simulink library "WellClearMetricsBlock"  (R2018b)
settings: Solver=VariableStepAuto  StartTime=0.0  StopTime=10.0  RelTol=1e-3
undefined symbols (not defined in the file): magnitude, wcm_altThresh, wcm_HMD, wcm_modTau, wcm_rangeThresh, wcm_TOCA
libraries: simulink x3
settings Model: Creator=BI28030  LastModifiedBy=BI28030

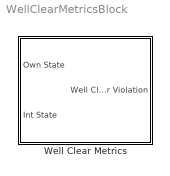
== system WellClearMetricsBlock ==
  Well Clear Metrics : Subsystem  mask{tauThreshold=wcm_modTau, hmdThreshold=wcm_HMD, tauVThreshold=wcm_TOCA, altThreshold=wcm_altThresh, rngThreshold=wcm_rangeThresh}
      mask prompts: tauThreshold "Modified Tau Threshold (s)"; hmdThreshold "Horizontal Miss Distance Threshold (ft)"; tauVThreshold "Time to Co-Altitude Threshold (s)"; altThreshold "Altitude Threshold (ft)"; rngThreshold "Range Threshold (ft)"
      mask help: Determines whether the intruder aircraft is within the bounds of a tau-based well clear region. Input is ownship and intruder 6-element state vectors in north, east, altitude coordinates. Returns true if a well-clear violation exists, false otherwise.

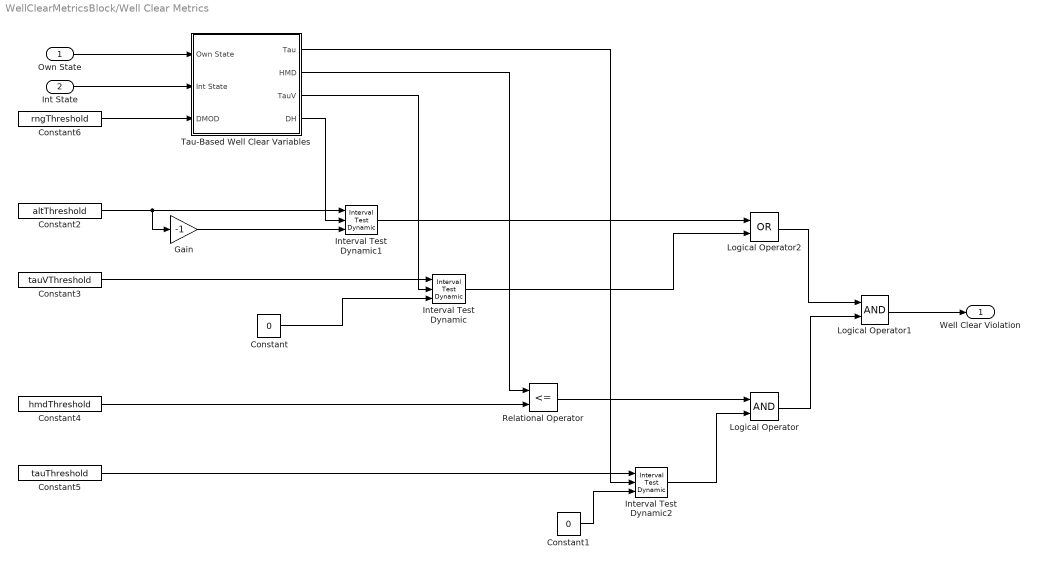
== system WellClearMetricsBlock/Well Clear Metrics ==
  Own State : Inport
  Int State : Inport  Port=2
  Constant : Constant  Value=0
  Constant1 : Constant  Value=0
  Constant2 : Constant  Value=altThreshold
  Constant3 : Constant  Value=tauVThreshold
  Constant4 : Constant  Value=hmdThreshold
  Constant5 : Constant  Value=tauThreshold
  Constant6 : Constant  Value=rngThreshold
  Gain : Gain  Gain=-1
  Interval Test Dynamic : simulink/Logic and Bit Operations/Interval Test Dynamic  IntervalClosedRight=on  IntervalClosedLeft=on  OutDataTypeStr=boolean
      settings: SourceProductName=Simulink  SourceProductBaseCode=SL
  Interval Test Dynamic1 : simulink/Logic and Bit Operations/Interval Test Dynamic  IntervalClosedRight=on  IntervalClosedLeft=on  OutDataTypeStr=boolean
      settings: SourceProductName=Simulink  SourceProductBaseCode=SL
  Interval Test Dynamic2 : simulink/Logic and Bit Operations/Interval Test Dynamic  IntervalClosedRight=on  IntervalClosedLeft=on  OutDataTypeStr=boolean
      settings: SourceProductName=Simulink  SourceProductBaseCode=SL
  Logical Operator : Logic  AllPortsSameDT=off  OutDataTypeStr=boolean
  Logical Operator1 : Logic  AllPortsSameDT=off  OutDataTypeStr=boolean
  Logical Operator2 : Logic  Operator=OR  AllPortsSameDT=off  OutDataTypeStr=boolean
  Relational Operator : RelationalOperator  Operator=<=  OutDataTypeStr=boolean  RndMeth=Nearest
  Tau-Based Well Clear Variables : Subsystem
  Well Clear Violation : Outport
  wires:
  Tau-Based Well Clear Variables/4(DH) -> Interval Test Dynamic1/2
  Tau-Based Well Clear Variables/3(TauV) -> Interval Test Dynamic/2
  Tau-Based Well Clear Variables/2(HMD) -> Relational Operator/1
  Relational Operator/1 -> Logical Operator/1
  Constant/1 -> Interval Test Dynamic/3
  Constant3/1 -> Interval Test Dynamic/1
  Int State/1 -> Tau-Based Well Clear Variables/2(Int State)
  Constant2/1 -> Gain/1, Interval Test Dynamic1/1
  Own State/1 -> Tau-Based Well Clear Variables/1(Own State)
  Logical Operator2/1 -> Logical Operator1/1
  Gain/1 -> Interval Test Dynamic1/3
  Constant1/1 -> Interval Test Dynamic2/3
  Constant5/1 -> Interval Test Dynamic2/1
  Tau-Based Well Clear Variables/1(Tau) -> Interval Test Dynamic2/2
  Interval Test Dynamic2/1 -> Logical Operator/2
  Interval Test Dynamic1/1 -> Logical Operator2/1
  Logical Operator1/1 -> Well Clear Violation/1
  Logical Operator/1 -> Logical Operator1/2
  Interval Test Dynamic/1 -> Logical Operator2/2
  Constant4/1 -> Relational Operator/2
  Constant6/1 -> Tau-Based Well Clear Variables/3(DMOD)

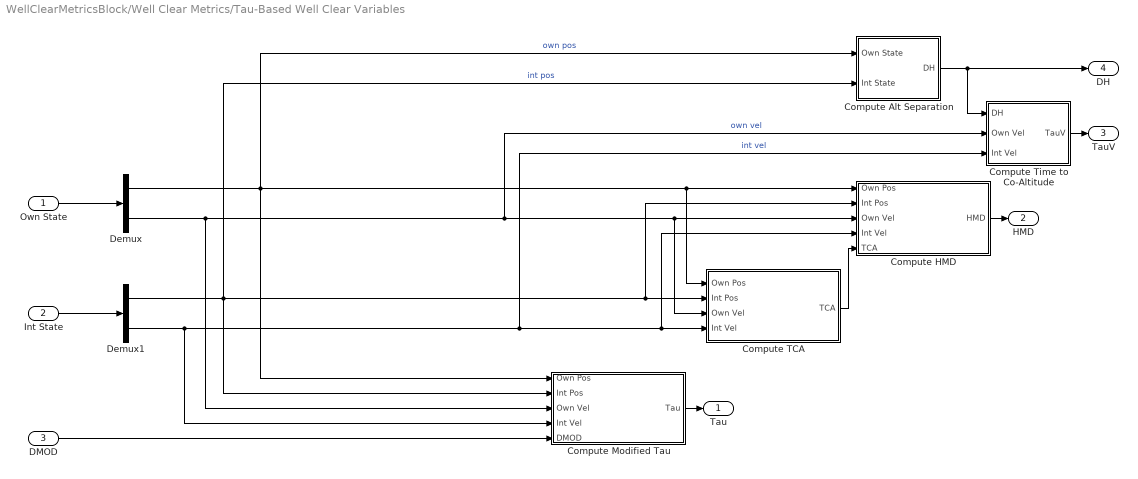
== system WellClearMetricsBlock/Well Clear Metrics/Tau-Based Well Clear Variables ==
  Own State : Inport
  Int State : Inport  Port=2
  DMOD : Inport  Port=3
  Compute Alt Separation : Subsystem
  Compute HMD : Subsystem
  Compute Modified Tau : Subsystem
  Compute TCA : Subsystem
  Compute Time to Co-Altitude : Subsystem
  Demux : Demux  Outputs=2
  Demux1 : Demux  Outputs=2
  Tau : Outport
  HMD : Outport  Port=2
  TauV : Outport  Port=3
  DH : Outport  Port=4
  wires:
  Demux1/1 -> Compute Alt Separation/2(Int State), Compute Modified Tau/2(Int Pos), Compute HMD/2(Int Pos), Compute TCA/2(Int Pos)  "int pos"
  Demux/1 -> Compute Alt Separation/1(Own State), Compute Modified Tau/1(Own Pos), Compute TCA/1(Own Pos), Compute HMD/1(Own Pos)  "own pos"
  Int State/1 -> Demux1/1
  Demux1/2 -> Compute Modified Tau/4(Int Vel), Compute Time to Co-Altitude/3(Int Vel), Compute HMD/4(Int Vel), Compute TCA/4(Int Vel)  "int vel"
  Demux/2 -> Compute Modified Tau/3(Own Vel), Compute Time to Co-Altitude/2(Own Vel), Compute TCA/3(Own Vel), Compute HMD/3(Own Vel)  "own vel"
  Compute Alt Separation/1(DH) -> DH/1, Compute Time to Co-Altitude/1(DH)
  Compute TCA/1(TCA) -> Compute HMD/5(TCA)
  Compute HMD/1(HMD) -> HMD/1
  Compute Time to Co-Altitude/1(TauV) -> TauV/1
  Compute Modified Tau/1(Tau) -> Tau/1
  Own State/1 -> Demux/1
  DMOD/1 -> Compute Modified Tau/5(DMOD)

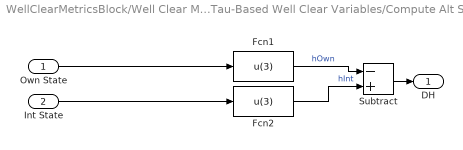
== system WellClearMetricsBlock/Well Clear Metrics/Tau-Based Well Clear Variables/Compute Alt Separation ==
  Own State : Inport
  Int State : Inport  Port=2
  Fcn1 : Fcn  Expr=u(3)
  Fcn2 : Fcn  Expr=u(3)
  Subtract : Sum  Inputs=-+
  DH : Outport
  wires:
  Subtract/1 -> DH/1
  Own State/1 -> Fcn1/1
  Int State/1 -> Fcn2/1
  Fcn2/1 -> Subtract/2  "hInt"
  Fcn1/1 -> Subtract/1  "hOwn"

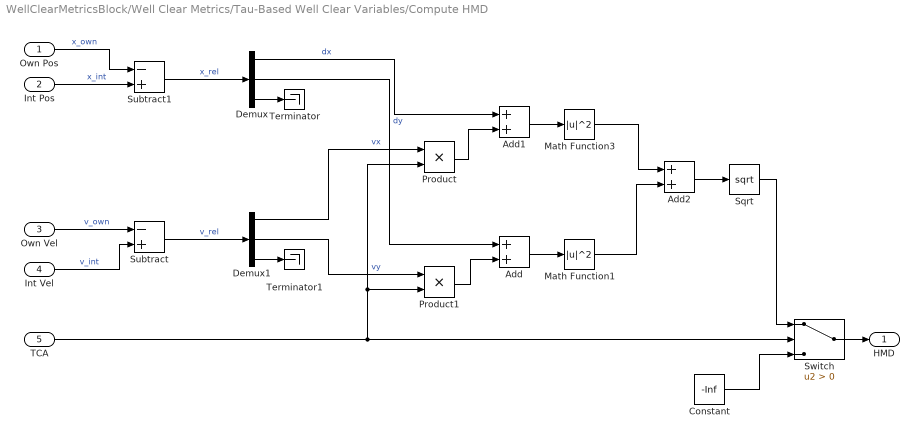
== system WellClearMetricsBlock/Well Clear Metrics/Tau-Based Well Clear Variables/Compute HMD ==
  Own Pos : Inport
  Int Pos : Inport  Port=2
  Own Vel : Inport  Port=3
  Int Vel : Inport  Port=4
  TCA : Inport  Port=5
  Add : Sum
  Add1 : Sum
  Add2 : Sum
  Constant : Constant  Value=-Inf
  Demux : Demux  Outputs=3
  Demux1 : Demux  Outputs=3
  Math Function1 : Math  Operator=magnitude^2  SaturateOnIntegerOverflow=on
  Math Function3 : Math  Operator=magnitude^2  SaturateOnIntegerOverflow=on
  Product : Product  RndMeth=Zero
  Product1 : Product  RndMeth=Zero
  Sqrt : Sqrt  SaturateOnIntegerOverflow=on
  Subtract : Sum  Inputs=-+
  Subtract1 : Sum  Inputs=-+
  Switch : Switch  Criteria=u2 > Threshold
  Terminator : Terminator
  Terminator1 : Terminator
  HMD : Outport
  wires:
  Int Vel/1 -> Subtract/2  "v_int"
  Int Pos/1 -> Subtract1/2  "x_int"
  Subtract1/1 -> Demux/1  "x_rel"
  Own Pos/1 -> Subtract1/1  "x_own"
  Own Vel/1 -> Subtract/1  "v_own"
  Subtract/1 -> Demux1/1  "v_rel"
  Demux1/1 -> Product/1  "vx"
  Demux1/2 -> Product1/1  "vy"
  Math Function3/1 -> Add2/1
  Add2/1 -> Sqrt/1
  Demux/1 -> Add1/1  "dx"
  Product/1 -> Add1/2
  TCA/1 -> Switch/2, Product1/2, Product/2
  Product1/1 -> Add/2
  Demux/2 -> Add/1  "dy"
  Add/1 -> Math Function1/1
  Add1/1 -> Math Function3/1
  Math Function1/1 -> Add2/2
  Sqrt/1 -> Switch/1
  Switch/1 -> HMD/1
  Constant/1 -> Switch/3
  Demux/3 -> Terminator/1
  Demux1/3 -> Terminator1/1

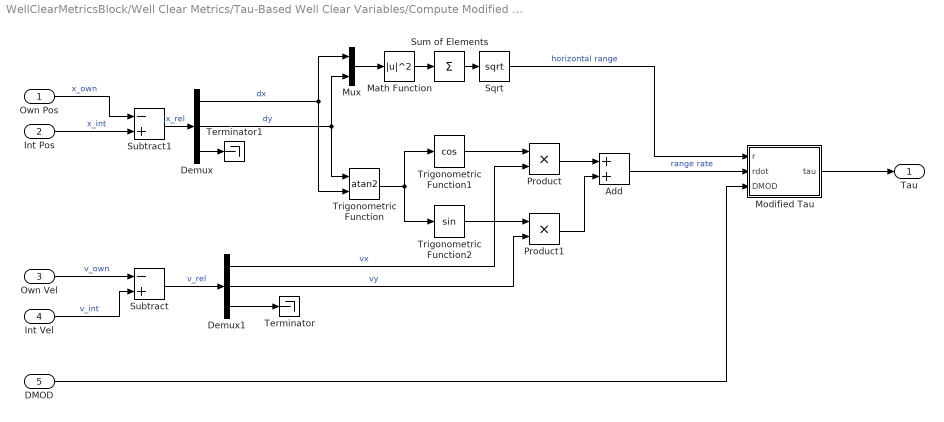
== system WellClearMetricsBlock/Well Clear Metrics/Tau-Based Well Clear Variables/Compute Modified Tau ==
  Own Pos : Inport
  Int Pos : Inport  Port=2
  Own Vel : Inport  Port=3
  Int Vel : Inport  Port=4
  DMOD : Inport  Port=5
  Add : Sum
  Demux : Demux  Outputs=3
  Demux1 : Demux  Outputs=3
  Math Function : Math  Operator=magnitude^2  SaturateOnIntegerOverflow=on
  Modified Tau : MATLAB Function  TreatAsAtomicUnit=on
  Mux : Mux  Inputs=2
  Product : Product  RndMeth=Zero
  Product1 : Product  RndMeth=Zero
  Sqrt : Sqrt  SaturateOnIntegerOverflow=on
  Subtract : Sum  Inputs=-+
  Subtract1 : Sum  Inputs=-+
  Sum of Elements : Sum  Inputs=+
  Terminator : Terminator
  Terminator1 : Terminator
  Trigonometric Function : Trigonometry  Operator=atan2
  Trigonometric Function1 : Trigonometry  Operator=cos
  Trigonometric Function2 : Trigonometry
  Tau : Outport
  wires:
  Mux/1 -> Math Function/1
  Demux/3 -> Terminator1/1
  Modified Tau/1(tau) -> Tau/1
  Math Function/1 -> Sum of Elements/1
  Sqrt/1 -> Modified Tau/1(r)  "horizontal range"
  Int Vel/1 -> Subtract/2  "v_int"
  Int Pos/1 -> Subtract1/2  "x_int"
  Subtract1/1 -> Demux/1  "x_rel"
  Own Pos/1 -> Subtract1/1  "x_own"
  Own Vel/1 -> Subtract/1  "v_own"
  Sum of Elements/1 -> Sqrt/1
  Demux/1 -> Trigonometric Function/2, Mux/1  "dx"
  Demux/2 -> Trigonometric Function/1, Mux/2  "dy"
  Add/1 -> Modified Tau/2(rdot)  "range rate"
  Trigonometric Function/1 -> Trigonometric Function1/1, Trigonometric Function2/1
  Product/1 -> Add/1
  Product1/1 -> Add/2
  Trigonometric Function2/1 -> Product1/1
  Trigonometric Function1/1 -> Product/1
  Subtract/1 -> Demux1/1  "v_rel"
  Demux1/1 -> Product/2  "vx"
  Demux1/2 -> Product1/2  "vy"
  DMOD/1 -> Modified Tau/3(DMOD)
  Demux1/3 -> Terminator/1

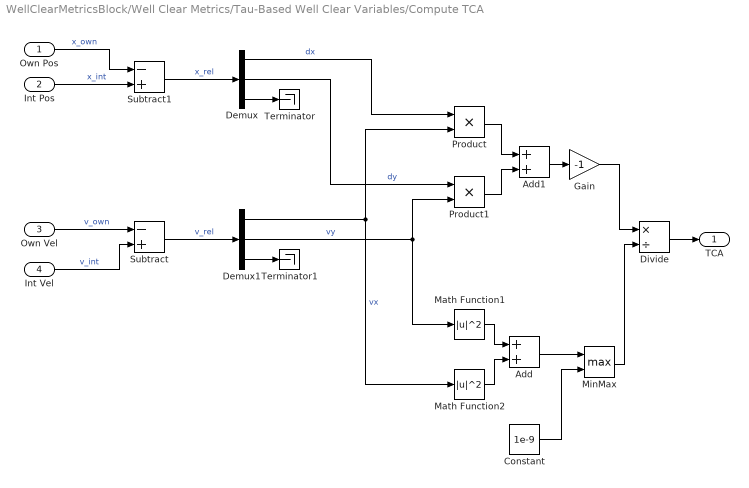
== system WellClearMetricsBlock/Well Clear Metrics/Tau-Based Well Clear Variables/Compute TCA ==
  Own Pos : Inport
  Int Pos : Inport  Port=2
  Own Vel : Inport  Port=3
  Int Vel : Inport  Port=4
  Add : Sum
  Add1 : Sum
  Constant : Constant  Value=1e-9
  Demux : Demux  Outputs=3
  Demux1 : Demux  Outputs=3
  Divide : Product  Inputs=*/
  Gain : Gain  Gain=-1
  Math Function1 : Math  Operator=magnitude^2  SaturateOnIntegerOverflow=on
  Math Function2 : Math  Operator=magnitude^2  SaturateOnIntegerOverflow=on
  MinMax : MinMax  Function=max  Inputs=2
  Product : Product  RndMeth=Zero
  Product1 : Product  RndMeth=Zero
  Subtract : Sum  Inputs=-+
  Subtract1 : Sum  Inputs=-+
  Terminator : Terminator
  Terminator1 : Terminator
  TCA : Outport
  wires:
  Divide/1 -> TCA/1
  Int Vel/1 -> Subtract/2  "v_int"
  Int Pos/1 -> Subtract1/2  "x_int"
  Subtract1/1 -> Demux/1  "x_rel"
  Own Pos/1 -> Subtract1/1  "x_own"
  Own Vel/1 -> Subtract/1  "v_own"
  Demux/1 -> Product/1  "dx"
  Demux/2 -> Product1/1  "dy"
  Subtract/1 -> Demux1/1  "v_rel"
  Demux1/1 -> Math Function2/1, Product/2  "vx"
  Demux1/2 -> Math Function1/1, Product1/2  "vy"
  Math Function1/1 -> Add/1
  Product/1 -> Add1/1
  Add/1 -> MinMax/1
  Math Function2/1 -> Add/2
  Product1/1 -> Add1/2
  Add1/1 -> Gain/1
  Gain/1 -> Divide/1
  Demux/3 -> Terminator/1
  Demux1/3 -> Terminator1/1
  MinMax/1 -> Divide/2
  Constant/1 -> MinMax/2

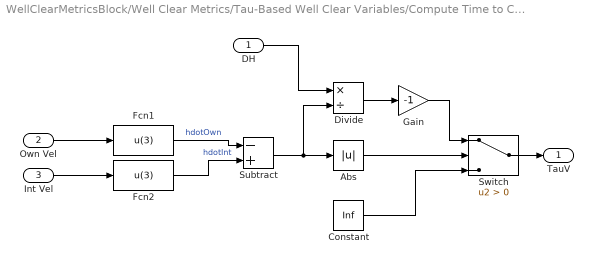
== system WellClearMetricsBlock/Well Clear Metrics/Tau-Based Well Clear Variables/Compute Time to Co-Altitude ==
  DH : Inport
  Own Vel : Inport  Port=2
  Int Vel : Inport  Port=3
  Abs : Abs
  Constant : Constant  Value=Inf
  Divide : Product  Inputs=*/
  Fcn1 : Fcn  Expr=u(3)
  Fcn2 : Fcn  Expr=u(3)
  Gain : Gain  Gain=-1
  Subtract : Sum  Inputs=-+
  Switch : Switch  Criteria=u2 > Threshold
  TauV : Outport
  wires:
  Constant/1 -> Switch/3
  Gain/1 -> Switch/1
  Abs/1 -> Switch/2
  Subtract/1 -> Divide/2, Abs/1
  Fcn1/1 -> Subtract/1  "hdotOwn"
  Divide/1 -> Gain/1
  Own Vel/1 -> Fcn1/1
  Fcn2/1 -> Subtract/2  "hdotInt"
  Int Vel/1 -> Fcn2/1
  Switch/1 -> TauV/1
  DH/1 -> Divide/1

== matlab function WellClearMetricsBlock/Well Clear Metrics/Tau-Based Well Clear Variables/Compute Modified Tau/Modified Tau ==
  data: r input; tau output; rdot input; DMOD input
function tau = fcn(r,rdot,DMOD)
%#codegen

if rdot >= 0 && r >= DMOD
  tau = Inf;
elseif r > DMOD
  tau = -(r^2 - DMOD^2)/(r*rdot);
else
  tau = 0;
end
